simulink subsystem "IMU"  (R2021a)
settings: Solver=VariableStepAuto  StartTime=0.0  StopTime=10.0  RelTol=1e-3
values from neighbouring files (symbols this model uses):
  misalignment = R_yaw*R_pitch*R_roll    [imu_params.m]
  Ts = 1/freq    (= 0.0005)    [imu_params.m]
undefined symbols (not defined in the file or in its folder): acc, gyro
libraries: simulink x8, dspsrcs4 x6
settings Model: Creator=Laura  LastModifiedBy=Laura

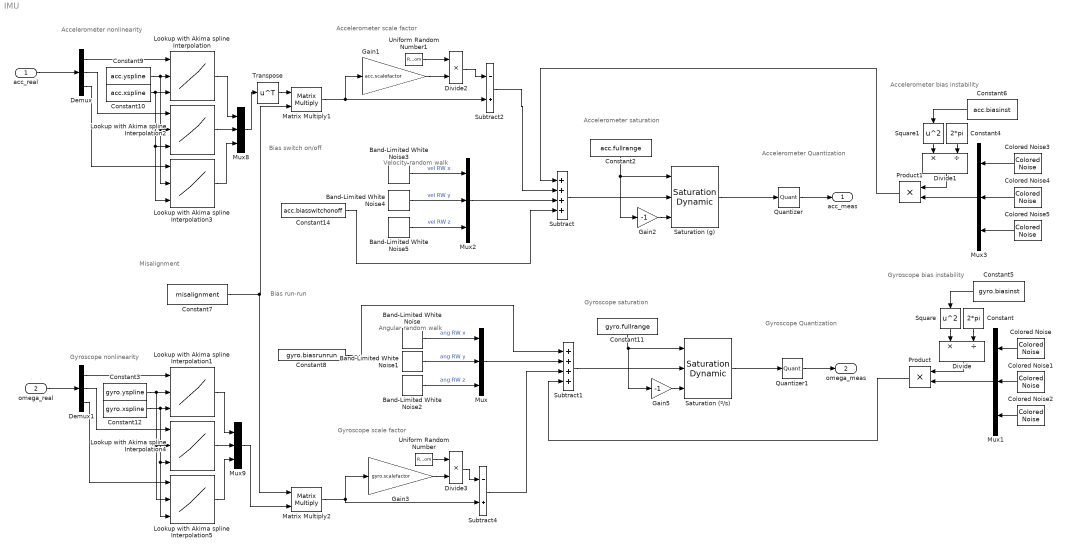
== system IMU ==
  note: Bias switch on/off
  note: Bias run-run
  note: Gyroscope saturation
  note: Gyroscope
      | Quantization
  note: Accelerometer
      | Quantization
  note: Gyroscope nonlinearity
  note: Accelerometer saturation
  note: Accelerometer scale factor
  note: Accelerometer nonlinearity
  note: Gyroscope scale factor
  note: Angular random walk
  note: Accelerometer bias instability
  note: Gyroscope bias instability
  note: Velocity random walk
  note: Misalignment
  acc_real : Inport
  omega_real : Inport  Port=2
  Band-Limited White Noise : simulink/Sources/Band-Limited White Noise  Cov=gyro.noisepower(1)  Ts=Ts  seed=[234234111]
  Band-Limited White Noise1 : simulink/Sources/Band-Limited White Noise  Cov=gyro.noisepower(2)  Ts=Ts  seed=[567380]
  Band-Limited White Noise2 : simulink/Sources/Band-Limited White Noise  Cov=gyro.noisepower(3)  Ts=Ts  seed=[3256]
  Band-Limited White Noise3 : simulink/Sources/Band-Limited White Noise  Cov=acc.noisepower(1)  Ts=Ts  seed=[32323556]
  Band-Limited White Noise4 : simulink/Sources/Band-Limited White Noise  Cov=acc.noisepower(2)  Ts=Ts  seed=[238641]
  Band-Limited White Noise5 : simulink/Sources/Band-Limited White Noise  Cov=acc.noisepower(3)  Ts=Ts  seed=[23341231]
  Colored Noise : dspsrcs4/Colored Noise  Color=pink  InverseFrequencyPower=1  BoundedOutput=off  NumChannels=1  OutputDataType=double  SamplesPerFrame=1  SampleTime=Ts  RandomStream=mt19937ar with seed  Seed=12237  SimulateUsing=Interpreted execution
      settings: SourceProductBaseCode=DS
  Colored Noise1 : dspsrcs4/Colored Noise  Color=pink  InverseFrequencyPower=1  BoundedOutput=off  NumChannels=1  OutputDataType=double  SamplesPerFrame=1  SampleTime=Ts  RandomStream=mt19937ar with seed  Seed=76372  SimulateUsing=Interpreted execution
      settings: SourceProductBaseCode=DS
  Colored Noise2 : dspsrcs4/Colored Noise  Color=pink  InverseFrequencyPower=1  BoundedOutput=off  NumChannels=1  OutputDataType=double  SamplesPerFrame=1  SampleTime=Ts  RandomStream=mt19937ar with seed  Seed=3755  SimulateUsing=Interpreted execution
      settings: SourceProductBaseCode=DS
  Colored Noise3 : dspsrcs4/Colored Noise  Color=pink  InverseFrequencyPower=1  BoundedOutput=off  NumChannels=1  OutputDataType=double  SamplesPerFrame=1  SampleTime=Ts  RandomStream=mt19937ar with seed  Seed=12237  SimulateUsing=Interpreted execution
      settings: SourceProductBaseCode=DS
  Colored Noise4 : dspsrcs4/Colored Noise  Color=pink  InverseFrequencyPower=1  BoundedOutput=off  NumChannels=1  OutputDataType=double  SamplesPerFrame=1  SampleTime=Ts  RandomStream=mt19937ar with seed  Seed=76372  SimulateUsing=Interpreted execution
      settings: SourceProductBaseCode=DS
  Colored Noise5 : dspsrcs4/Colored Noise  Color=pink  InverseFrequencyPower=1  BoundedOutput=off  NumChannels=1  OutputDataType=double  SamplesPerFrame=1  SampleTime=Ts  RandomStream=mt19937ar with seed  Seed=3755  SimulateUsing=Interpreted execution
      settings: SourceProductBaseCode=DS
  Constant : Constant  Value=2*pi
  Constant10 : Constant  Value=acc.xspline
  Constant11 : Constant  Value=gyro.fullrange
  Constant12 : Constant  Value=gyro.xspline
  Constant14 : Constant  Value=acc.biasswitchonoff
  Constant2 : Constant  Value=acc.fullrange
  Constant3 : Constant  Value=gyro.yspline
  Constant4 : Constant  Value=2*pi
  Constant5 : Constant  Value=gyro.biasinst
  Constant6 : Constant  Value=acc.biasinst
  Constant7 : Constant  Value=misalignment
  Constant8 : Constant  Value=gyro.biasrunrun
  Constant9 : Constant  Value=acc.yspline
  Demux : Demux  Outputs=3
  Demux1 : Demux  Outputs=3
  Divide : Product  Inputs=*/
  Divide1 : Product  Inputs=*/
  Divide2 : Product  Inputs=**
  Divide3 : Product  Inputs=**
  Gain1 : Gain  Gain=acc.scalefactor
  Gain2 : Gain  Gain=-1
  Gain3 : Gain  Gain=gyro.scalefactor
  Gain5 : Gain  Gain=-1
  Lookup with Akima spline Interpolation{,1..5} (6 alike) : Lookup_n-D  NumberOfTableDimensions=1  BreakpointsForDimension1Source=Input port  BreakpointsForDimension1=[-5:5]  TableSource=Input port  Table=tanh([-5:5])  InterpMethod=Cubic spline  InternalRulePriority=Speed  RndMeth=Simplest  InputSameDT=on
      settings: InputPortMap=u0,p221,p5
  Matrix Multiply1 : Product  Multiplication=Matrix(*)
  Matrix Multiply2 : Product  Multiplication=Matrix(*)
  Mux{,1..3,8..9} (6 alike) : Mux  Inputs=3
  Product : Product
  Product1 : Product
  Quantizer : Quantizer  QuantizationInterval=acc.quantization
  Quantizer1 : Quantizer  QuantizationInterval=gyro.quantization
  Saturation (g) : simulink/Discontinuities/Saturation Dynamic  OutMin=[]  OutMax=[]  OutDataTypeStr=Inherit: Same as second input  OutDataType=fixdt(1, 16)  OutScaling=2^-10  DoSatur=off
  Saturation (º/s) : simulink/Discontinuities/Saturation Dynamic  OutMin=[]  OutMax=[]  OutDataTypeStr=Inherit: Same as second input  OutDataType=fixdt(1, 16)  OutScaling=2^-10  DoSatur=off
  Square : Math  Operator=square  SaturateOnIntegerOverflow=on
  Square1 : Math  Operator=square  SaturateOnIntegerOverflow=on
  Subtract : Sum  Inputs=++++
  Subtract1 : Sum  Inputs=++++
  Subtract2 : Sum  Inputs=-+
  Subtract4 : Sum  Inputs=-+
  Transpose : Math  Operator=transpose  SaturateOnIntegerOverflow=on
  Uniform Random Number : UniformRandomNumber  SampleTime=0.005
  Uniform Random Number1 : UniformRandomNumber  SampleTime=0.005
  acc_meas : Outport  SampleTime=Ts
  omega_meas : Outport  Port=2  SampleTime=Ts
  wires:
  Colored Noise2/1 -> Mux1/3
  Band-Limited White Noise1/1 -> Mux/2  "ang RW y"
  Band-Limited White Noise5/1 -> Mux2/3  "vel RW z"
  Band-Limited White Noise4/1 -> Mux2/2  "vel RW y"
  Constant5/1 -> Square/1
  Mux2/1 -> Subtract/3
  Band-Limited White Noise3/1 -> Mux2/1  "vel RW x"
  Square/1 -> Divide/1
  Colored Noise1/1 -> Mux1/2
  Band-Limited White Noise/1 -> Mux/1  "ang RW x"
  Constant/1 -> Divide/2
  Band-Limited White Noise2/1 -> Mux/3  "ang RW z"
  Colored Noise/1 -> Mux1/1
  Colored Noise4/1 -> Mux3/2
  Colored Noise3/1 -> Mux3/1
  Colored Noise5/1 -> Mux3/3
  Square1/1 -> Divide1/1
  Constant6/1 -> Square1/1
  Constant4/1 -> Divide1/2
  Mux3/1 -> Product1/2
  Divide1/1 -> Product1/1
  Product1/1 -> Subtract/1
  Quantizer1/1 -> omega_meas/1
  Divide/1 -> Product/1
  Mux1/1 -> Product/2
  Constant10/1 -> Lookup with Akima spline Interpolation/3, Lookup with Akima spline Interpolation2/3, Lookup with Akima spline Interpolation3/3
  Constant9/1 -> Lookup with Akima spline Interpolation/2, Lookup with Akima spline Interpolation2/2, Lookup with Akima spline Interpolation3/2
  Matrix Multiply1/1 -> Subtract2/2, Gain1/1
  Subtract2/1 -> Subtract/2
  Gain2/1 -> Saturation (g)/3
  Constant2/1 -> Gain2/1, Saturation (g)/1
  Saturation (º/s)/1 -> Quantizer1/1
  Constant11/1 -> Saturation (º/s)/1, Gain5/1
  Gain5/1 -> Saturation (º/s)/3
  Subtract1/1 -> Saturation (º/s)/2
  Quantizer/1 -> acc_meas/1
  Subtract4/1 -> Subtract1/3
  Divide3/1 -> Subtract4/1
  Uniform Random Number/1 -> Divide3/1
  Gain3/1 -> Divide3/2
  Matrix Multiply2/1 -> Gain3/1, Subtract4/2
  Constant7/1 -> Matrix Multiply2/1, Matrix Multiply1/2
  acc_real/1 -> Demux/1
  Lookup with Akima spline Interpolation2/1 -> Mux8/2
  Lookup with Akima spline Interpolation/1 -> Mux8/1
  Lookup with Akima spline Interpolation3/1 -> Mux8/3
  Demux/1 -> Lookup with Akima spline Interpolation/1
  Demux/2 -> Lookup with Akima spline Interpolation2/1
  Demux/3 -> Lookup with Akima spline Interpolation3/1
  Transpose/1 -> Matrix Multiply1/1
  Mux8/1 -> Transpose/1
  omega_real/1 -> Demux1/1
  Lookup with Akima spline Interpolation1/1 -> Mux9/1
  Lookup with Akima spline Interpolation4/1 -> Mux9/2
  Lookup with Akima spline Interpolation5/1 -> Mux9/3
  Demux1/1 -> Lookup with Akima spline Interpolation1/1
  Constant3/1 -> Lookup with Akima spline Interpolation1/2, Lookup with Akima spline Interpolation4/2, Lookup with Akima spline Interpolation5/2
  Constant12/1 -> Lookup with Akima spline Interpolation1/3, Lookup with Akima spline Interpolation4/3, Lookup with Akima spline Interpolation5/3
  Demux1/2 -> Lookup with Akima spline Interpolation4/1
  Demux1/3 -> Lookup with Akima spline Interpolation5/1
  Mux9/1 -> Matrix Multiply2/2
  Uniform Random Number1/1 -> Divide2/1
  Gain1/1 -> Divide2/2
  Divide2/1 -> Subtract2/1
  Constant14/1 -> Subtract/4
  Mux/1 -> Subtract1/2
  Product/1 -> Subtract1/4
  Constant8/1 -> Subtract1/1
  Subtract/1 -> Saturation (g)/2
  Saturation (g)/1 -> Quantizer/1
